simulink model "VehicleDynamicsModel"  (R2018a)
settings: Solver=ode15s  StartTime=0.0  StopTime=12  FixedStep=0.01  RelTol=1e-2  EnableMultiTasking=on
PreLoadFcn:
  | PowerTrain_14DOF_ini
StopFcn:
  | AfterSim
undefined symbols (not defined in the file): AccelCmd2TrqCmd, Chasis, GearRatio, Motor, Motor_J, Motor_RotorDamping, VEH, X, Y, Z
libraries: sm_lib x186, autolibutils x40, nesl_utility x23, vehdynlibtire x4, fuzblock x3, sharedtransform x2, autolibmappedmotorcommon x2, vehdynlibeom x1, vehdynlibsuspension x1, simulink x1, vehdynlibsteering x1
(part 7 of 11)

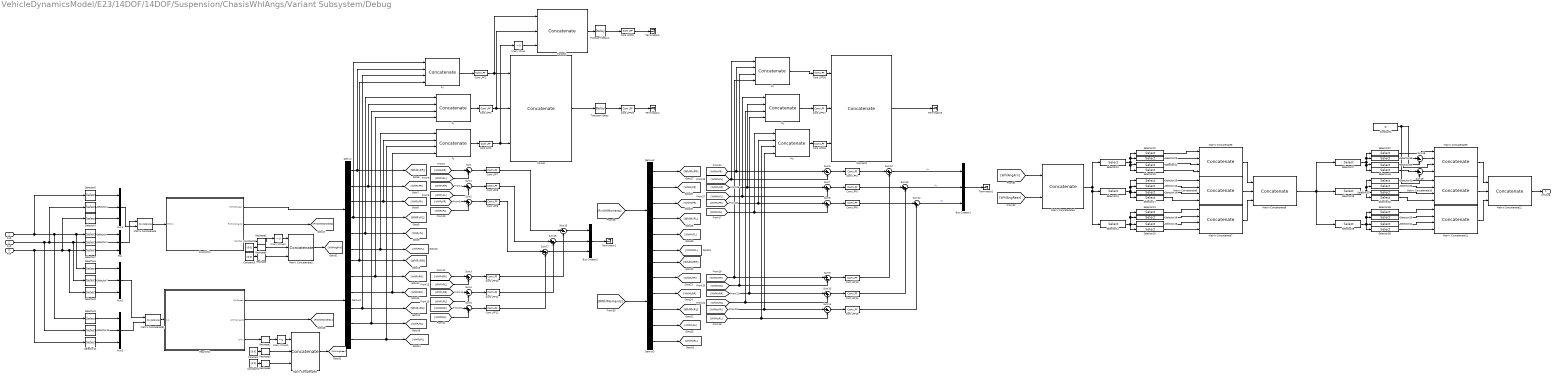
== system VehicleDynamicsModel/E23/14DOF/14DOF/Suspension/ChasisWhlAngs/Variant Subsystem/Debug ==
  FxR : Inport
  FyR : Inport  Port=2
  FzR : Inport  Port=3
  Bus Creator1 : BusCreator  Inputs=3
  Bus Creator2 : BusCreator  Inputs=3
  Constant{,1..3} (4 alike) : Constant  Value=[0 0]
  Constant4 : Constant  Value=pi
  Cont LPF{1..20} (20 alike) : autolibutils/Cont LPF  wc=2*pi  aMode=2
      settings: SourceProductName=Powertrain Blockset  SourceProductBaseCode=PW
  Demux{,1..3} (4 alike) : Demux  Outputs=6
  Forces : Concatenate  NumInputs=3  Mode=Multidimensional array
  Forces1 : Concatenate  NumInputs=3  Mode=Multidimensional array
  FrontWhls : Subsystem  TreatAsAtomicUnit=on
  Fx : Concatenate  NumInputs=4  Mode=Multidimensional array  ConcatenateDimension=2
  Fy : Concatenate  NumInputs=4  Mode=Multidimensional array  ConcatenateDimension=2
  Fz : Concatenate  NumInputs=4  Mode=Multidimensional array  ConcatenateDimension=2
  Matrix Concatenate : Concatenate  Mode=Multidimensional array  ConcatenateDimension=2
  Matrix Concatenate1 : Concatenate  Mode=Multidimensional array  ConcatenateDimension=2
  Matrix Concatenate{5..7,9..11} (6 alike) : Concatenate  NumInputs=4  Mode=Multidimensional array  ConcatenateDimension=2
  Matrix Concatenate{2..3,8,12} (4 alike) : Concatenate  NumInputs=3  Mode=Multidimensional array
  Matrix Concatenate4 : Concatenate  Mode=Multidimensional array  ConcatenateDimension=2
  Moments : Concatenate  NumInputs=3  Mode=Multidimensional array
  Mux{,1..3} (4 alike) : Mux  Inputs=3
  Mx : Concatenate  NumInputs=4  Mode=Multidimensional array  ConcatenateDimension=2
  My : Concatenate  NumInputs=4  Mode=Multidimensional array  ConcatenateDimension=2
  Mz : Concatenate  NumInputs=4  Mode=Multidimensional array  ConcatenateDimension=2
  RearWhls : Subsystem  TreatAsAtomicUnit=on
  Reshape{,1..5} (6 alike) : Reshape  OutputDimensionality=Row vector (2-D)
  Selector{,1..2,21..22,26,36..37,41} (9 alike) : Selector  InputPortWidth=4  IndexOptions=Index vector (dialog)  Indices=1  OutputSizes=1
  Selector{9..11,17,20,25,32,35,40} (9 alike) : Selector  InputPortWidth=4  IndexOptions=Index vector (dialog)  Indices=4  OutputSizes=1
  Selector12 : Selector  NumberOfDimensions=2  InputPortWidth=3  IndexOptions=Index vector (dialog),Select all  Indices=1,1  OutputSizes=1,1
  Selector13 : Selector  NumberOfDimensions=2  InputPortWidth=3  IndexOptions=Index vector (dialog),Select all  Indices=2,1  OutputSizes=1,1
  Selector14 : Selector  NumberOfDimensions=2  InputPortWidth=3  IndexOptions=Index vector (dialog),Select all  Indices=3,1  OutputSizes=1,1
  Selector{3..5,15,18,23,30,33,38} (9 alike) : Selector  InputPortWidth=4  IndexOptions=Index vector (dialog)  Indices=2  OutputSizes=1
  Selector{6..8,16,19,24,31,34,39} (9 alike) : Selector  InputPortWidth=4  IndexOptions=Index vector (dialog)  Indices=3  OutputSizes=1
  Selector27 : Selector  NumberOfDimensions=2  InputPortWidth=3  IndexOptions=Index vector (dialog),Select all  Indices=1,1  OutputSizes=1,1
  Selector28 : Selector  NumberOfDimensions=2  InputPortWidth=3  IndexOptions=Index vector (dialog),Select all  Indices=2,1  OutputSizes=1,1
  Selector29 : Selector  NumberOfDimensions=2  InputPortWidth=3  IndexOptions=Index vector (dialog),Select all  Indices=3,1  OutputSizes=1,1
  Sum{,2..3,5,7,10,12..14,16..17} (11 alike) : Sum  Inputs=|++
  Sum{1,4,6,8..9,11,15,18..19} (9 alike) : Sum  Inputs=|+-
  Terminator{1..5} (5 alike) : Terminator
  Transport Delay : TransportDelay  DelayTime=0
  Transport Delay1 : TransportDelay  DelayTime=0
  Unary Minus : UnaryMinus
  Unary Minus1 : UnaryMinus
  Unary Minus2 : UnaryMinus
  WhlAng : Outport
  wires:
  Matrix Concatenate7/1 -> Matrix Concatenate8/3
  Matrix Concatenate5/1 -> Matrix Concatenate8/1
  FyR/1 -> Selector10/1, Selector4/1, Selector7/1, Selector1/1
  FzR/1 -> Selector11/1, Selector3/1, Selector8/1, Selector2/1
  Selector17/1 -> Matrix Concatenate6/4
  Selector16/1 -> Matrix Concatenate6/3
  Matrix Concatenate4/1 -> Selector14/1, Selector13/1, Selector12/1
  Selector15/1 -> Matrix Concatenate6/2
  Selector21/1 -> Matrix Concatenate7/1
  Matrix Concatenate8/1 -> Selector29/1, Selector27/1, Selector28/1
  Selector40/1 -> Sum19/1
  Selector39/1 -> Matrix Concatenate9/3
  Sum19/1 -> Matrix Concatenate9/4
  Selector13/1 -> Selector15/1, Selector26/1, Selector17/1, Selector16/1
  Selector12/1 -> Selector25/1, Selector24/1, Selector23/1, Selector22/1
  Selector14/1 -> Selector20/1, Selector19/1, Selector18/1, Selector21/1
  Selector22/1 -> Matrix Concatenate5/1
  Selector37/1 -> Matrix Concatenate9/1
  Matrix Concatenate11/1 -> Matrix Concatenate12/3
  Selector36/1 -> Matrix Concatenate11/1
  Selector28/1 -> Selector30/1, Selector41/1, Selector32/1, Selector31/1
  Selector38/1 -> Sum18/1
  Selector27/1 -> Selector40/1, Selector39/1, Selector38/1, Selector37/1
  Matrix Concatenate10/1 -> Matrix Concatenate12/2
  Selector31/1 -> Matrix Concatenate10/3
  Selector32/1 -> Matrix Concatenate10/4
  Matrix Concatenate9/1 -> Matrix Concatenate12/1
  Constant4/1 -> Sum19/2, Sum18/2
  Selector34/1 -> Matrix Concatenate11/3
  Selector30/1 -> Matrix Concatenate10/2
  Sum18/1 -> Matrix Concatenate9/2
  Matrix Concatenate12/1 -> WhlAng/1
  [WhlMzRL] -> Mz/3, Sum11/2
  [WhlMxRL] -> Mx/3, Sum9/2
  [RWhlMoments] -> Demux3/1
  Demux1/2 -> Fy/4, [WhlFyRR]
  [WhlMyFL] -> My/1, Sum7/2
  Bus Creator2/1 -> Terminator1/1
  Mux2/1 -> Matrix Concatenate1/1
  Cont LPF6/1 -> Sum14/1
  Demux2/5 -> [WhlMyFL]
  [WhlMxFR] -> Mx/2, Sum6/1
  Selector33/1 -> Matrix Concatenate11/2
  My/1 -> Cont LPF17/1
  [WhlMyFR] -> My/2, Sum7/1
  Demux1/3 -> Fz/4, [WhlFzRR]
  Sum2/1 -> Cont LPF9/1
  Selector4/1 -> Mux1/2
  Demux/4 -> Fx/1, [WhlFxFL]
  Sum7/1 -> Cont LPF5/1
  Demux2/1 -> [WhlMxFR]
  RearWhls/1(WhlForces) -> Demux1/1
  Fy/1 -> Cont LPF1/1
  Matrix Concatenate1/1 -> RearWhls/1(In1)
  Demux3/2 -> [WhlMyRR]
  Moments/1 -> Terminator5/1
  Demux3/1 -> [WhlMxRR]
  [WhlFxRL] -> Sum3/2
  Reshape/1 -> Matrix Concatenate2/3
  Demux1/5 -> Fy/3, [WhlFyRL]
  FrontWhls/1(FWhlsForces) -> Demux/1
  [WhlFzFR] -> Sum2/1
  Demux2/6 -> [WhlMzFL]
  Cont LPF11/1 -> Sum16/2
  Sum1/1 -> Cont LPF8/1
  Cont LPF8/1 -> Sum16/1
  Demux1/1 -> Fx/4, [WhlFxRR]
  Sum17/1 -> Bus Creator2/3
  [WhlFyRL] -> Sum4/2
  [WhlMyRL] -> My/3, Sum10/2
  Selector24/1 -> Matrix Concatenate5/3
  Selector6/1 -> Mux2/1
  Cont LPF1/1 -> Forces1/2, Forces/2
  Cont LPF10/1 -> Sum15/2
  Demux3/4 -> [WhlMxRL]
  Cont LPF3/1 -> Unary Minus/1, Forces/3
  Cont LPF7/1 -> Sum15/1
  Cont LPF15/1 -> Sum14/2
  Sum4/1 -> Cont LPF11/1
  Mx/1 -> Cont LPF16/1
  [WhlFyFR] -> Sum1/1
  [WhlFzRR] -> Sum5/1
  Mux3/1 -> Matrix Concatenate1/2
  Cont LPF17/1 -> Moments/2
  Sum5/1 -> Cont LPF12/1
  Cont LPF2/1 -> Forces1/1, Forces/1
  [WhlFyRR] -> Sum4/1
  Selector26/1 -> Matrix Concatenate6/1
  Selector10/1 -> Mux3/2
  Unary Minus/1 -> Forces1/3
  [WhlFxRR] -> Sum3/1
  Forces/1 -> Transport Delay/1
  Transport Delay/1 -> Cont LPF19/1
  Selector8/1 -> Mux2/3
  Demux2/2 -> [WhlMyFR]
  Reshape4/1 -> Matrix Concatenate2/2
  Sum10/1 -> Cont LPF14/1
  Matrix Concatenate3/1 -> [WhlAngRear]
  Cont LPF9/1 -> Sum17/1
  [WhlAngFrn] -> Matrix Concatenate4/1
  Sum14/1 -> Bus Creator1/3  "Mz"
  Cont LPF19/1 -> Terminator4/1
  Cont LPF20/1 -> Terminator3/1
  Cont LPF16/1 -> Moments/1
  Demux/5 -> Fy/1, [WhlFyFL]
  Selector29/1 -> Selector35/1, Selector34/1, Selector33/1, Selector36/1
  RearWhls/2(WhlMoments) -> [RWhlMoments]
  Selector1/1 -> Mux/2
  Mux/1 -> Matrix Concatenate/1
  [WhlMxFL] -> Sum6/2, Mx/1
  [WhlFxFL] -> Sum/2
  Selector5/1 -> Mux1/1
  Constant/1 -> Reshape3/1
  Matrix Concatenate/1 -> FrontWhls/1(FWhls)
  Cont LPF5/1 -> Sum13/1
  Demux2/4 -> [WhlMxFL]
  Sum8/1 -> Cont LPF6/1
  Demux3/3 -> [WhlMzRR]
  Selector9/1 -> Mux3/1
  Selector11/1 -> Mux3/3
  Mux1/1 -> Matrix Concatenate/2
  Reshape2/1 -> Unary Minus1/1
  [WhlFzRL] -> Sum5/2
  Demux1/6 -> Fz/3, [WhlFzRL]
  Bus Creator1/1 -> Terminator2/1
  Selector23/1 -> Matrix Concatenate5/2
  Selector35/1 -> Matrix Concatenate11/4
  Constant3/1 -> Reshape/1
  RearWhls/3(Whl1) -> Reshape2/1
  Constant2/1 -> Reshape4/1
  Reshape5/1 -> Matrix Concatenate3/3
  Reshape3/1 -> Matrix Concatenate3/2
  Demux2/3 -> [WhlMzFR]
  Selector20/1 -> Matrix Concatenate7/4
  Selector18/1 -> Matrix Concatenate7/2
  Forces1/1 -> Transport Delay1/1
  Constant1/1 -> Reshape5/1
  FrontWhls/2(FWhlMoments) -> [FrnWhlMoments]
  Sum/1 -> Cont LPF7/1
  Demux3/6 -> [WhlMzRL]
  FrontWhls/3(Camber) -> Reshape1/1
  Reshape1/1 -> Unary Minus2/1
  Unary Minus1/1 -> Matrix Concatenate3/1
  Selector3/1 -> Mux1/3
  Demux3/5 -> [WhlMyRL]
  Selector41/1 -> Matrix Concatenate10/1
  Sum13/1 -> Bus Creator1/2  "My"
  Selector19/1 -> Matrix Concatenate7/3
  [WhlMzRR] -> Mz/4, Sum11/1
  Matrix Concatenate2/1 -> [WhlAngFrn]
  Cont LPF12/1 -> Sum17/2
  Cont LPF13/1 -> Sum12/2
  [WhlMzFR] -> Mz/2, Sum8/1
  Demux/3 -> Fz/2, [WhlFzFR]
  Demux/1 -> Fx/2, [WhlFxFR]
  [FrnWhlMoments] -> Demux2/1
  Demux/2 -> Fy/2, [WhlFyFR]
  Sum11/1 -> Cont LPF15/1
  Cont LPF18/1 -> Moments/3
  Sum12/1 -> Bus Creator1/1  "Mx"
  Sum15/1 -> Bus Creator2/1
  Cont LPF14/1 -> Sum13/2
  Fz/1 -> Cont LPF3/1
  Transport Delay1/1 -> Cont LPF20/1
  Sum9/1 -> Cont LPF13/1
  [WhlMxRR] -> Mx/4, Sum9/1
  Mz/1 -> Cont LPF18/1
  [WhlAngRear] -> Matrix Concatenate4/2
  [WhlMzFL] -> Mz/1, Sum8/2
  [WhlFzFL] -> Sum2/2
  [WhlFxFR] -> Sum/1
  Fx/1 -> Cont LPF2/1
  Selector/1 -> Mux/1
  Selector7/1 -> Mux2/2
  [WhlFyFL] -> Sum1/2
  Sum3/1 -> Cont LPF10/1
  Demux1/4 -> Fx/3, [WhlFxRL]
  Matrix Concatenate6/1 -> Matrix Concatenate8/2
  Selector2/1 -> Mux/3
  Sum16/1 -> Bus Creator2/2
  [WhlMyRR] -> My/4, Sum10/1
  Sum6/1 -> Cont LPF4/1
  Unary Minus2/1 -> Matrix Concatenate2/1
  Selector25/1 -> Matrix Concatenate5/4
  Demux/6 -> Fz/1, [WhlFzFL]
  Cont LPF4/1 -> Sum12/1
  FxR/1 -> Selector5/1, Selector9/1, Selector6/1, Selector/1

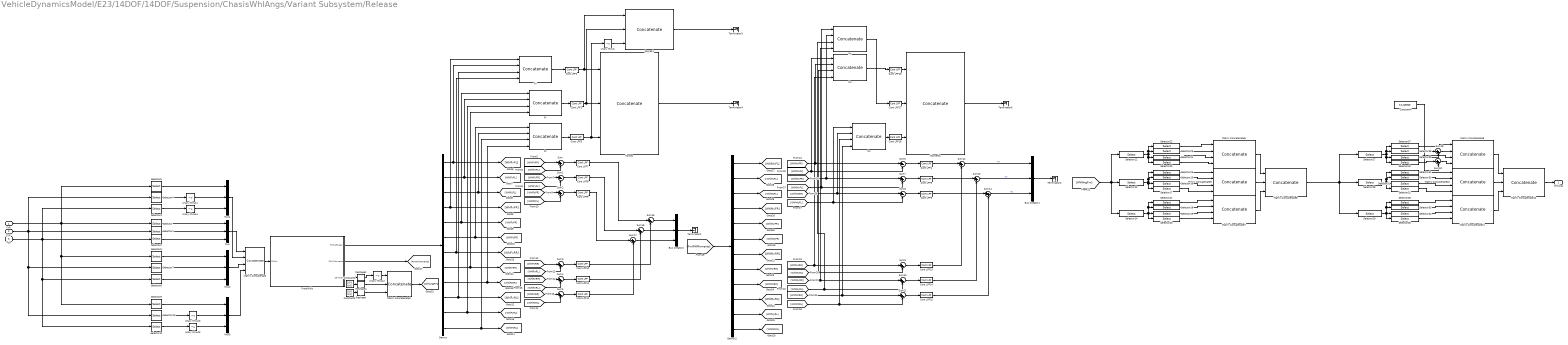
== system VehicleDynamicsModel/E23/14DOF/14DOF/Suspension/ChasisWhlAngs/Variant Subsystem/Release ==
  FxR : Inport
  FyR : Inport  Port=2
  FzR : Inport  Port=3
  Bus Creator1 : BusCreator  Inputs=3
  Bus Creator2 : BusCreator  Inputs=3
  Constant2 : Constant  Value=[0 0 0 0]
  Constant3 : Constant  Value=[0 0 0 0]
  Constant4 : Constant  Value=3.1415926
  Cont LPF{1..18} (18 alike) : autolibutils/Cont LPF  wc=2*pi  aMode=2
      settings: SourceProductName=Powertrain Blockset  SourceProductBaseCode=PW
  Demux : Demux  Outputs=12
  Demux2 : Demux  Outputs=12
  Forces : Concatenate  NumInputs=3  Mode=Multidimensional array
  Forces1 : Concatenate  NumInputs=3  Mode=Multidimensional array
  FrontWhls : Subsystem  TreatAsAtomicUnit=on
  Fx : Concatenate  NumInputs=4  Mode=Multidimensional array  ConcatenateDimension=2
  Fy : Concatenate  NumInputs=4  Mode=Multidimensional array  ConcatenateDimension=2
  Fz : Concatenate  NumInputs=4  Mode=Multidimensional array  ConcatenateDimension=2
  Matrix Concatenate{,5..7,9..11} (7 alike) : Concatenate  NumInputs=4  Mode=Multidimensional array  ConcatenateDimension=2
  Matrix Concatenate12 : Concatenate  NumInputs=3  Mode=Multidimensional array
  Matrix Concatenate2 : Concatenate  NumInputs=3  Mode=Multidimensional array
  Matrix Concatenate8 : Concatenate  NumInputs=3  Mode=Multidimensional array
  Moments : Concatenate  NumInputs=3  Mode=Multidimensional array
  Mux{,1..3} (4 alike) : Mux  Inputs=3
  Mx : Concatenate  NumInputs=4  Mode=Multidimensional array  ConcatenateDimension=2
  My : Concatenate  NumInputs=4  Mode=Multidimensional array  ConcatenateDimension=2
  Mz : Concatenate  NumInputs=4  Mode=Multidimensional array  ConcatenateDimension=2
  Reshape : Reshape  OutputDimensionality=Row vector (2-D)
  Reshape1 : Reshape  OutputDimensionality=Row vector (2-D)
  Reshape4 : Reshape  OutputDimensionality=Row vector (2-D)
  Selector{,1..2,21..22,26,36..37,41} (9 alike) : Selector  InputPortWidth=4  IndexOptions=Index vector (dialog)  Indices=1  OutputSizes=1
  Selector{9..11,17,20,25,32,35,40} (9 alike) : Selector  InputPortWidth=4  IndexOptions=Index vector (dialog)  Indices=4  OutputSizes=1
  Selector12 : Selector  NumberOfDimensions=2  InputPortWidth=3  IndexOptions=Index vector (dialog),Select all  Indices=1,1  OutputSizes=1,1
  Selector13 : Selector  NumberOfDimensions=2  InputPortWidth=3  IndexOptions=Index vector (dialog),Select all  Indices=2,1  OutputSizes=1,1
  Selector14 : Selector  NumberOfDimensions=2  InputPortWidth=3  IndexOptions=Index vector (dialog),Select all  Indices=3,1  OutputSizes=1,1
  Selector{3..5,15,18,23,30,33,38} (9 alike) : Selector  InputPortWidth=4  IndexOptions=Index vector (dialog)  Indices=2  OutputSizes=1
  Selector{6..8,16,19,24,31,34,39} (9 alike) : Selector  InputPortWidth=4  IndexOptions=Index vector (dialog)  Indices=3  OutputSizes=1
  Selector27 : Selector  NumberOfDimensions=2  InputPortWidth=3  IndexOptions=Index vector (dialog),Select all  Indices=1,1  OutputSizes=1,1
  Selector28 : Selector  NumberOfDimensions=2  InputPortWidth=3  IndexOptions=Index vector (dialog),Select all  Indices=2,1  OutputSizes=1,1
  Selector29 : Selector  NumberOfDimensions=2  InputPortWidth=3  IndexOptions=Index vector (dialog),Select all  Indices=3,1  OutputSizes=1,1
  Sum{,2..3,5,7,10,12..14,16..17} (11 alike) : Sum  Inputs=|++
  Sum{1,4,6,8..9,11,15,18..19} (9 alike) : Sum  Inputs=|+-
  Terminator{1..5} (5 alike) : Terminator
  Unary Minus{,1..5} (6 alike) : UnaryMinus
  WhlAng : Outport
  wires:
  Matrix Concatenate7/1 -> Matrix Concatenate8/3
  Matrix Concatenate5/1 -> Matrix Concatenate8/1
  FyR/1 -> Selector7/1, Selector10/1, Selector1/1, Selector4/1
  FzR/1 -> Selector3/1, Selector11/1, Selector8/1, Selector2/1
  Selector17/1 -> Matrix Concatenate6/4
  Selector16/1 -> Matrix Concatenate6/3
  [WhlAngFrn] -> Selector12/1, Selector14/1, Selector13/1
  Selector15/1 -> Matrix Concatenate6/2
  Selector21/1 -> Matrix Concatenate7/1
  Matrix Concatenate8/1 -> Selector29/1, Selector27/1, Selector28/1
  Selector13/1 -> Selector15/1, Selector26/1, Selector17/1, Selector16/1
  Selector12/1 -> Selector25/1, Selector24/1, Selector23/1, Selector22/1
  Selector14/1 -> Selector20/1, Selector19/1, Selector18/1, Selector21/1
  Selector22/1 -> Matrix Concatenate5/1
  Selector37/1 -> Matrix Concatenate9/1
  Matrix Concatenate11/1 -> Matrix Concatenate12/3
  Selector36/1 -> Matrix Concatenate11/1
  Selector28/1 -> Selector30/1, Selector41/1, Selector32/1, Selector31/1
  Selector38/1 -> Sum18/1
  Selector27/1 -> Selector40/1, Selector39/1, Selector38/1, Selector37/1
  Matrix Concatenate10/1 -> Matrix Concatenate12/2
  Selector31/1 -> Matrix Concatenate10/3
  Selector32/1 -> Matrix Concatenate10/4
  Matrix Concatenate9/1 -> Matrix Concatenate12/1
  Constant4/1 -> Sum18/2, Sum19/2
  Selector34/1 -> Matrix Concatenate11/3
  Selector30/1 -> Matrix Concatenate10/2
  Sum18/1 -> Matrix Concatenate9/2
  Matrix Concatenate12/1 -> WhlAng/1
  [WhlMzRL] -> Mz/3, Sum11/2
  [WhlMxRL] -> Mx/3, Sum9/2
  Demux/8 -> Fy/4, [WhlFyRR]
  [WhlMyFL] -> My/1, Sum7/2
  Bus Creator2/1 -> Terminator1/1
  Mux2/1 -> Matrix Concatenate/3
  Cont LPF6/1 -> Sum14/1
  Demux2/5 -> [WhlMyFR]
  [WhlMxFR] -> Mx/2, Sum6/1
  Selector33/1 -> Matrix Concatenate11/2
  My/1 -> Cont LPF17/1
  [WhlMyFR] -> My/2, Sum7/1
  Demux/9 -> Fz/4, [WhlFzRR]
  Sum2/1 -> Cont LPF9/1
  Selector4/1 -> Unary Minus1/1
  Demux/4 -> Fx/1, [WhlFxFR]
  Sum7/1 -> Cont LPF5/1
  Demux2/1 -> [WhlMxFL]
  Fy/1 -> Cont LPF1/1
  Demux2/8 -> [WhlMyRR]
  Moments/1 -> Terminator5/1
  Demux2/7 -> [WhlMxRR]
  [WhlFxRL] -> Sum3/2
  Reshape/1 -> Matrix Concatenate2/3
  Demux/11 -> Fy/3, [WhlFyRL]
  FrontWhls/1(FWhlsForces) -> Demux/1
  [WhlFzFR] -> Sum2/1
  Demux2/6 -> [WhlMzFR]
  Cont LPF11/1 -> Sum16/2
  Sum1/1 -> Cont LPF8/1
  Cont LPF8/1 -> Sum16/1
  Demux/7 -> Fx/4, [WhlFxRR]
  Sum17/1 -> Bus Creator2/3
  [WhlFyRL] -> Sum4/2
  [WhlMyRL] -> My/3, Sum10/2
  Selector24/1 -> Matrix Concatenate5/3
  Selector6/1 -> Mux2/1
  Cont LPF1/1 -> Forces1/2, Forces/2
  Cont LPF10/1 -> Sum15/2
  Demux2/10 -> [WhlMxRL]
  Cont LPF3/1 -> Unary Minus/1, Forces/3
  Cont LPF7/1 -> Sum15/1
  Cont LPF15/1 -> Sum14/2
  Sum4/1 -> Cont LPF11/1
  Mx/1 -> Cont LPF16/1
  [WhlFyFR] -> Sum1/1
  [WhlFzRR] -> Sum5/1
  Mux3/1 -> Matrix Concatenate/4
  Cont LPF17/1 -> Moments/2
  Sum5/1 -> Cont LPF12/1
  Cont LPF2/1 -> Forces1/1, Forces/1
  [WhlFyRR] -> Sum4/1
  Selector26/1 -> Matrix Concatenate6/1
  Unary Minus/1 -> Forces1/3
  [WhlFxRR] -> Sum3/1
  Demux2/2 -> [WhlMyFL]
  Reshape4/1 -> Matrix Concatenate2/2
  Sum10/1 -> Cont LPF14/1
  Cont LPF9/1 -> Sum17/1
  Sum14/1 -> Bus Creator1/3  "Mz"
  Forces/1 -> Terminator4/1
  Forces1/1 -> Terminator3/1
  Cont LPF16/1 -> Moments/1
  Demux/5 -> Fy/1, [WhlFyFR]
  Selector29/1 -> Selector35/1, Selector34/1, Selector33/1, Selector36/1
  [WhlMxFL] -> Sum6/2, Mx/1
  [WhlFxFL] -> Sum/2
  Matrix Concatenate/1 -> FrontWhls/1(FWhls)
  Cont LPF5/1 -> Sum13/1
  Demux2/4 -> [WhlMxFR]
  Sum8/1 -> Cont LPF6/1
  Demux2/9 -> [WhlMzRR]
  Selector9/1 -> Mux3/1
  [WhlFzRL] -> Sum5/2
  Demux/12 -> Fz/3, [WhlFzRL]
  Bus Creator1/1 -> Terminator2/1
  Selector23/1 -> Matrix Concatenate5/2
  Selector35/1 -> Matrix Concatenate11/4
  Constant3/1 -> Reshape/1
  Constant2/1 -> Reshape4/1
  Demux2/3 -> [WhlMzFL]
  Selector20/1 -> Matrix Concatenate7/4
  Selector18/1 -> Matrix Concatenate7/2
  FrontWhls/2(FWhlMoments) -> [FrnWhlMoments]
  Sum/1 -> Cont LPF7/1
  Demux2/12 -> [WhlMzRL]
  Reshape1/1 -> Unary Minus2/1
  Demux2/11 -> [WhlMyRL]
  Selector41/1 -> Matrix Concatenate10/1
  Sum13/1 -> Bus Creator1/2  "My"
  Selector19/1 -> Matrix Concatenate7/3
  [WhlMzRR] -> Mz/4, Sum11/1
  Matrix Concatenate2/1 -> [WhlAngFrn]
  Cont LPF12/1 -> Sum17/2
  Cont LPF13/1 -> Sum12/2
  [WhlMzFR] -> Mz/2, Sum8/1
  Demux/3 -> Fz/2, [WhlFzFL]
  Demux/1 -> Fx/2, [WhlFxFL]
  [FrnWhlMoments] -> Demux2/1
  Demux/2 -> Fy/2, [WhlFyFL]
  Sum11/1 -> Cont LPF15/1
  Cont LPF18/1 -> Moments/3
  Sum12/1 -> Bus Creator1/1  "Mx"
  Sum15/1 -> Bus Creator2/1
  Cont LPF14/1 -> Sum13/2
  Fz/1 -> Cont LPF3/1
  Sum9/1 -> Cont LPF13/1
  [WhlMxRR] -> Mx/4, Sum9/1
  Mz/1 -> Cont LPF18/1
  [WhlMzFL] -> Mz/1, Sum8/2
  [WhlFzFL] -> Sum2/2
  [WhlFxFR] -> Sum/1
  Fx/1 -> Cont LPF2/1
  Selector/1 -> Mux/1
  Selector7/1 -> Mux2/2
  [WhlFyFL] -> Sum1/2
  Sum3/1 -> Cont LPF10/1
  Demux/10 -> Fx/3, [WhlFxRL]
  Matrix Concatenate6/1 -> Matrix Concatenate8/2
  Sum16/1 -> Bus Creator2/2
  [WhlMyRR] -> Sum10/1, My/4
  Sum6/1 -> Cont LPF4/1
  Unary Minus2/1 -> Matrix Concatenate2/1
  Selector25/1 -> Matrix Concatenate5/4
  Demux/6 -> Fz/1, [WhlFzFR]
  Cont LPF4/1 -> Sum12/1
  FxR/1 -> Selector6/1, Selector9/1, Selector/1, Selector5/1
  Selector39/1 -> Matrix Concatenate9/3
  Selector40/1 -> Sum19/1
  Sum19/1 -> Matrix Concatenate9/4
  Mux/1 -> Matrix Concatenate/1
  Mux1/1 -> Matrix Concatenate/2
  Selector5/1 -> Mux1/1
  Selector3/1 -> Unary Minus4/1
  Selector8/1 -> Mux2/3
  Selector11/1 -> Unary Minus5/1
  Selector2/1 -> Mux/3
  FrontWhls/3(Camber) -> Reshape1/1
  Selector10/1 -> Unary Minus3/1
  Selector1/1 -> Mux/2
  Unary Minus3/1 -> Mux3/2
  Unary Minus1/1 -> Mux1/2
  Unary Minus4/1 -> Mux1/3
  Unary Minus5/1 -> Mux3/3

== system VehicleDynamicsModel/E23/14DOF/14DOF/Tires&Wheels/VDBS/4Wheels/Fx ==
  In1 : Inport
  In2 : Inport  Port=2
  In3 : Inport  Port=3
  In4 : Inport  Port=4
  Bus Selector{,1..3} (4 alike) : BusSelector  OutputSignals=Fx
  Vector Concatenate : Concatenate  NumInputs=4
  Fx : Outport
  wires:
  Bus Selector/1 -> Vector Concatenate/1  "<Fx>"
  Bus Selector1/1 -> Vector Concatenate/2  "<Fx>"
  In2/1 -> Bus Selector1/1
  Vector Concatenate/1 -> Fx/1
  Bus Selector3/1 -> Vector Concatenate/4  "<Fx>"
  In3/1 -> Bus Selector2/1
  In4/1 -> Bus Selector3/1
  Bus Selector2/1 -> Vector Concatenate/3  "<Fx>"
  In1/1 -> Bus Selector/1

== system VehicleDynamicsModel/E23/14DOF/14DOF/Tires&Wheels/VDBS/4Wheels/Fy ==
  In1 : Inport
  In2 : Inport  Port=2
  In3 : Inport  Port=3
  In4 : Inport  Port=4
  Bus Selector{,1..3} (4 alike) : BusSelector  OutputSignals=Fy
  Vector Concatenate : Concatenate  NumInputs=4
  Fy : Outport
  wires:
  Bus Selector/1 -> Vector Concatenate/1  "<Fy>"
  Bus Selector1/1 -> Vector Concatenate/2  "<Fy>"
  In2/1 -> Bus Selector1/1
  Vector Concatenate/1 -> Fy/1
  Bus Selector3/1 -> Vector Concatenate/4  "<Fy>"
  In3/1 -> Bus Selector2/1
  In4/1 -> Bus Selector3/1
  Bus Selector2/1 -> Vector Concatenate/3  "<Fy>"
  In1/1 -> Bus Selector/1

== system VehicleDynamicsModel/E23/14DOF/14DOF/Tires&Wheels/VDBS/4Wheels/Fz ==
  In1 : Inport
  In2 : Inport  Port=2
  In3 : Inport  Port=3
  In4 : Inport  Port=4
  Bus Selector{,1..3} (4 alike) : BusSelector  OutputSignals=Fz
  Vector Concatenate : Concatenate  NumInputs=4
  Fz : Outport
  wires:
  Bus Selector/1 -> Vector Concatenate/1  "<Fz>"
  Bus Selector1/1 -> Vector Concatenate/2  "<Fz>"
  In2/1 -> Bus Selector1/1
  Vector Concatenate/1 -> Fz/1
  Bus Selector3/1 -> Vector Concatenate/4  "<Fz>"
  In3/1 -> Bus Selector2/1
  In4/1 -> Bus Selector3/1
  Bus Selector2/1 -> Vector Concatenate/3  "<Fz>"
  In1/1 -> Bus Selector/1

== system VehicleDynamicsModel/E23/14DOF/14DOF/Tires&Wheels/VDBS/4Wheels/Kappa ==
  In1 : Inport
  In2 : Inport  Port=2
  In3 : Inport  Port=3
  In4 : Inport  Port=4
  Bus Selector{,1..3} (4 alike) : BusSelector  OutputSignals=Kappa
  Vector Concatenate : Concatenate  NumInputs=4
  Kappa : Outport
  wires:
  Bus Selector/1 -> Vector Concatenate/1  "<Kappa>"
  Bus Selector1/1 -> Vector Concatenate/2  "<Kappa>"
  In2/1 -> Bus Selector1/1
  Vector Concatenate/1 -> Kappa/1
  Bus Selector3/1 -> Vector Concatenate/4  "<Kappa>"
  In3/1 -> Bus Selector2/1
  In4/1 -> Bus Selector3/1
  Bus Selector2/1 -> Vector Concatenate/3  "<Kappa>"
  In1/1 -> Bus Selector/1

== system VehicleDynamicsModel/E23/14DOF/14DOF/Tires&Wheels/VDBS/4Wheels/Mx ==
  In1 : Inport
  In2 : Inport  Port=2
  In3 : Inport  Port=3
  In4 : Inport  Port=4
  Bus Selector{,1..3} (4 alike) : BusSelector  OutputSignals=Mx
  Vector Concatenate : Concatenate  NumInputs=4
  Mx : Outport
  wires:
  Bus Selector/1 -> Vector Concatenate/1  "<Mx>"
  Bus Selector1/1 -> Vector Concatenate/2  "<Mx>"
  In2/1 -> Bus Selector1/1
  Vector Concatenate/1 -> Mx/1
  Bus Selector3/1 -> Vector Concatenate/4  "<Mx>"
  In3/1 -> Bus Selector2/1
  In4/1 -> Bus Selector3/1
  Bus Selector2/1 -> Vector Concatenate/3  "<Mx>"
  In1/1 -> Bus Selector/1

== system VehicleDynamicsModel/E23/14DOF/14DOF/Tires&Wheels/VDBS/4Wheels/My ==
  In1 : Inport
  In2 : Inport  Port=2
  In3 : Inport  Port=3
  In4 : Inport  Port=4
  Bus Selector{,1..3} (4 alike) : BusSelector  OutputSignals=My
  Vector Concatenate : Concatenate  NumInputs=4
  My : Outport
  wires:
  Bus Selector/1 -> Vector Concatenate/1  "<My>"
  Bus Selector1/1 -> Vector Concatenate/2  "<My>"
  In2/1 -> Bus Selector1/1
  Vector Concatenate/1 -> My/1
  Bus Selector3/1 -> Vector Concatenate/4  "<My>"
  In3/1 -> Bus Selector2/1
  In4/1 -> Bus Selector3/1
  Bus Selector2/1 -> Vector Concatenate/3  "<My>"
  In1/1 -> Bus Selector/1

== system VehicleDynamicsModel/E23/14DOF/14DOF/Tires&Wheels/VDBS/4Wheels/Mz ==
  In1 : Inport
  In2 : Inport  Port=2
  In3 : Inport  Port=3
  In4 : Inport  Port=4
  Bus Selector{,1..3} (4 alike) : BusSelector  OutputSignals=Mz
  Vector Concatenate : Concatenate  NumInputs=4
  Mz : Outport
  wires:
  Bus Selector/1 -> Vector Concatenate/1  "<Mz>"
  Bus Selector1/1 -> Vector Concatenate/2  "<Mz>"
  In2/1 -> Bus Selector1/1
  Vector Concatenate/1 -> Mz/1
  Bus Selector3/1 -> Vector Concatenate/4  "<Mz>"
  In3/1 -> Bus Selector2/1
  In4/1 -> Bus Selector3/1
  Bus Selector2/1 -> Vector Concatenate/3  "<Mz>"
  In1/1 -> Bus Selector/1

== system VehicleDynamicsModel/E23/14DOF/14DOF/Tires&Wheels/VDBS/4Wheels/Re ==
  In1 : Inport
  In2 : Inport  Port=2
  In3 : Inport  Port=3
  In4 : Inport  Port=4
  Bus Selector{,1..3} (4 alike) : BusSelector  OutputSignals=Re
  Vector Concatenate : Concatenate  NumInputs=4
  Re : Outport
  wires:
  Bus Selector/1 -> Vector Concatenate/1  "<Re>"
  Bus Selector1/1 -> Vector Concatenate/2  "<Re>"
  In2/1 -> Bus Selector1/1
  Vector Concatenate/1 -> Re/1
  Bus Selector3/1 -> Vector Concatenate/4  "<Re>"
  In3/1 -> Bus Selector2/1
  In4/1 -> Bus Selector3/1
  Bus Selector2/1 -> Vector Concatenate/3  "<Re>"
  In1/1 -> Bus Selector/1

== system VehicleDynamicsModel/E23/14DOF/14DOF/Tires&Wheels/VDBS/4Wheels/omega ==
  In1 : Inport
  In2 : Inport  Port=2
  In3 : Inport  Port=3
  In4 : Inport  Port=4
  Bus Selector{,1..3} (4 alike) : BusSelector  OutputSignals=Omega
  Vector Concatenate : Concatenate  NumInputs=4
  omege : Outport
  wires:
  Bus Selector/1 -> Vector Concatenate/1  "<Omega>"
  Bus Selector1/1 -> Vector Concatenate/2  "<Omega>"
  In2/1 -> Bus Selector1/1
  Vector Concatenate/1 -> omege/1
  Bus Selector3/1 -> Vector Concatenate/4  "<Omega>"
  In3/1 -> Bus Selector2/1
  In4/1 -> Bus Selector3/1
  Bus Selector2/1 -> Vector Concatenate/3  "<Omega>"
  In1/1 -> Bus Selector/1

== system VehicleDynamicsModel/E23/14DOF/14DOF/Tires&Wheels/VDBS/4Wheels/z ==
  In1 : Inport
  In2 : Inport  Port=2
  In3 : Inport  Port=3
  In4 : Inport  Port=4
  Bus Selector{,1..3} (4 alike) : BusSelector  OutputSignals=z
  Vector Concatenate : Concatenate  NumInputs=4
  Z : Outport
  wires:
  Bus Selector/1 -> Vector Concatenate/1  "<z>"
  Bus Selector1/1 -> Vector Concatenate/2  "<z>"
  In2/1 -> Bus Selector1/1
  Vector Concatenate/1 -> Z/1
  Bus Selector3/1 -> Vector Concatenate/4  "<z>"
  In3/1 -> Bus Selector2/1
  In4/1 -> Bus Selector3/1
  Bus Selector2/1 -> Vector Concatenate/3  "<z>"
  In1/1 -> Bus Selector/1

== system VehicleDynamicsModel/E23/14DOF/14DOF/Tires&Wheels/VDBS/4Wheels/zdot ==
  In1 : Inport
  In2 : Inport  Port=2
  In3 : Inport  Port=3
  In4 : Inport  Port=4
  Bus Selector{,1..3} (4 alike) : BusSelector  OutputSignals=zdot
  Vector Concatenate : Concatenate  NumInputs=4
  zdot : Outport
  wires:
  Bus Selector/1 -> Vector Concatenate/1  "<zdot>"
  Bus Selector1/1 -> Vector Concatenate/2  "<zdot>"
  In2/1 -> Bus Selector1/1
  Vector Concatenate/1 -> zdot/1
  Bus Selector3/1 -> Vector Concatenate/4  "<zdot>"
  In3/1 -> Bus Selector2/1
  In4/1 -> Bus Selector3/1
  Bus Selector2/1 -> Vector Concatenate/3  "<zdot>"
  In1/1 -> Bus Selector/1

== system VehicleDynamicsModel/E23/14DOF/14DOF/Tires&Wheels/VDBS/Tires2Veh/Subsystem ==
  note: 按行放置，即X ; Y ; Z
  note: 车轮坐标系
  note: 转向角（绕Z轴）
  note: 轮胎与车轮
      | 坐标系绕y轴
      | 角度为0
  note: 内倾角（绕X轴）
  Front : Inport
  Camber : Inport  Port=2
  Add : Sum
  Add1 : Sum
  Constant : Constant  Value=pi
  Constant1 : Constant  Value=[pi;0;pi;0].*0+[0;pi;0;pi].*.0
  Constant2 : Constant  Value=ones(1,4).*0
  Reshape : Reshape  OutputDimensionality=Row vector (2-D)
  Reshape1 : Reshape  OutputDimensionality=Row vector (2-D)
  Reshape2 : Reshape  OutputDimensionality=Row vector (2-D)
  Vector Concatenate1 : Concatenate  NumInputs=3  Mode=Multidimensional array
  Vehicle : Outport
  wires:
  Reshape/1 -> Vector Concatenate1/1
  Vector Concatenate1/1 -> Vehicle/1
  Add1/1 -> Reshape2/1
  Front/1 -> Add1/1
  Reshape1/1 -> Vector Concatenate1/2
  Constant1/1 -> Add1/2
  Reshape2/1 -> Vector Concatenate1/3
  Camber/1 -> Add/1
  Constant/1 -> Add/2
  Constant2/1 -> Reshape1/1
  Add/1 -> Reshape/1

== system VehicleDynamicsModel/E23/14DOF/14DOF/Tires&Wheels/VDBS/Tires2Veh/Subsystem1 ==
  Mx : Inport
  My : Inport  Port=2
  Mz : Inport  Port=3
  Re : Inport  Port=4
  z : Inport  Port=5
  zdot : Inport  Port=6
  Kappa : Inport  Port=7
  Fx : Inport  Port=8
  omega : Inport  Port=9
  Fy : Inport  Port=10
  Fz : Inport  Port=11
  Bus Creator : BusCreator  Inputs=11
  Reshape : Reshape  OutputDimensionality=Row vector (2-D)
  Reshape1 : Reshape  OutputDimensionality=Row vector (2-D)
  Unary Minus : UnaryMinus
  Unary Minus2 : UnaryMinus
  Whl : Outport
  zout : Outport  Port=2
  zdotout : Outport  Port=3
  wires:
  Mz/1 -> Bus Creator/7
  Fz/1 -> Bus Creator/4
  Fx/1 -> Bus Creator/2
  My/1 -> Bus Creator/6
  Fy/1 -> Bus Creator/3
  Re/1 -> Bus Creator/8
  omega/1 -> Bus Creator/1
  Mx/1 -> Bus Creator/5
  Unary Minus/1 -> Reshape1/1, Bus Creator/10  "zdot"
  Reshape1/1 -> zdotout/1
  Kappa/1 -> Bus Creator/11
  Bus Creator/1 -> Whl/1
  Reshape/1 -> zout/1
  Unary Minus2/1 -> Bus Creator/9, Reshape/1  "z"
  z/1 -> Unary Minus2/1  "z"
  zdot/1 -> Unary Minus/1

== system VehicleDynamicsModel/E23/14DOF/14DOF/Tires&Wheels/VDBS/Tires2Veh/WheeltoBodyTransform ==
  note: 矩阵相乘，把车轮坐标系下的力变换为车身坐标系下的力
  Forces : Inport  Partition=on  PartitionDimension=2  PartitionWidth=1  PartitionOffset=0
  WheelAngles : Inport  Port=2  Partition=on  PartitionDimension=2  PartitionWidth=1  PartitionOffset=0
  Demux : Demux  Outputs=3
  For Each : ForEach  DisableCoverage=on  IndexMode=One-based
  Matrix Multiply : Product  Multiplication=Matrix(*)
  Rotation Angles to Direction Cosine Matrix : sharedtransform/Rotation Angles to Direction Cosine Matrix  rotationOrder=ZYX  aMode=aMode
      settings: SourceProductBaseCode=AE
  Selector : Selector  InputPortWidth=3  IndexOptions=Index vector (dialog)  Indices=[3 2 1]  OutputSizes=1
  Fx : Outport  ConcatenationDimension=1
  Fy : Outport  Port=2  ConcatenationDimension=1
  Fz : Outport  Port=3  ConcatenationDimension=1
  wires:
  WheelAngles/1 -> Selector/1
  Selector/1 -> Rotation Angles to Direction Cosine Matrix/1
  Rotation Angles to Direction Cosine Matrix/1 -> Matrix Multiply/1
  Forces/1 -> Matrix Multiply/2
  Demux/1 -> Fx/1
  Matrix Multiply/1 -> Demux/1
  Demux/2 -> Fy/1
  Demux/3 -> Fz/1

== system VehicleDynamicsModel/E23/14DOF/14DOF/Tires&Wheels/VDBS/Veh2Tire/WheelAngles ==
  Camber : Inport
  Steer : Inport  Port=2
  Constant : Constant  Value=pi
  Constant2 : Constant  Value=[pi;0;pi;0].*0+[0;pi;0;pi].*0
  Reshape : Reshape  OutputDimensionality=Row vector (2-D)
  Reshape1 : Reshape  OutputDimensionality=Row vector (2-D)
  Reshape2 : Reshape  OutputDimensionality=Row vector (2-D)
  Vector Concatenate : Concatenate  NumInputs=3  Mode=Multidimensional array
  X : Sum
  Y : Constant  Value=ones(1,4).*0
  Z : Sum
  Vehicle : Outport
  wires:
  Y/1 -> Reshape1/1
  Reshape2/1 -> Vector Concatenate/3
  Constant/1 -> X/2
  Reshape1/1 -> Vector Concatenate/2
  Steer/1 -> Z/1
  Reshape/1 -> Vector Concatenate/1
  Vector Concatenate/1 -> Vehicle/1
  Camber/1 -> X/1
  Constant2/1 -> Z/2
  X/1 -> Reshape/1
  Z/1 -> Reshape2/1

== system VehicleDynamicsModel/E23/14DOF/14DOF/Tires&Wheels/VDBS/Veh2Tire/WheeltoBodyTransform ==
  note: 把车辆质心在车身坐标系下的速度转化为在车轮坐标系下的速度
  WheelAngles : Inport  Partition=on  PartitionDimension=2  PartitionWidth=1  PartitionOffset=0
  VelVeh : Inport  Port=2  Partition=on  PartitionDimension=2  PartitionWidth=1  PartitionOffset=0
  Demux : Demux  Outputs=3
  For Each : ForEach  DisableCoverage=on  IndexMode=One-based
  Matrix Multiply : Product  Multiplication=Matrix(*)
  Rotation Angles to Direction Cosine Matrix : sharedtransform/Rotation Angles to Direction Cosine Matrix  rotationOrder=ZYX  aMode=aMode
      settings: SourceProductBaseCode=AE
  Selector : Selector  InputPortWidth=3  IndexOptions=Index vector (dialog)  Indices=[3 2 1]  OutputSizes=1
  xdotWheel : Outport  ConcatenationDimension=1
  ydotWheel : Outport  Port=2  ConcatenationDimension=1
  zdotWheel : Outport  Port=3  ConcatenationDimension=1
  wires:
  WheelAngles/1 -> Selector/1
  Selector/1 -> Rotation Angles to Direction Cosine Matrix/1
  Rotation Angles to Direction Cosine Matrix/1 -> Matrix Multiply/1
  VelVeh/1 -> Matrix Multiply/2
  Matrix Multiply/1 -> Demux/1
  Demux/1 -> xdotWheel/1
  Demux/2 -> ydotWheel/1
  Demux/3 -> zdotWheel/1

== system VehicleDynamicsModel/E23/PowerTrain/PowerTrain/MotorRL/Motor/Motor/Mapped Motor ==
  BattVolt : Inport
  MtrSpd : Inport  Port=2
  TrqCmd : Inport  Port=3
  Mapped Motor Core Speed 4 : autolibmappedmotorcommon/Mapped Motor Core Speed 4
      settings: SourceProductName=Powertrain Blockset  SourceProductBaseCode=PW
  Info : Outport
  BattCurr : Outport  Port=2
  MtrTrq : Outport  Port=3
  wires:
  BattVolt/1 -> Mapped Motor Core Speed 4/1
  TrqCmd/1 -> Mapped Motor Core Speed 4/3
  MtrSpd/1 -> Mapped Motor Core Speed 4/2
  Mapped Motor Core Speed 4/2 -> BattCurr/1
  Mapped Motor Core Speed 4/1 -> Info/1
  Mapped Motor Core Speed 4/3 -> MtrTrq/1

== system VehicleDynamicsModel/E23/PowerTrain/PowerTrain/MotorRR/Motor/Motor/Mapped Motor ==
  BattVolt : Inport
  MtrSpd : Inport  Port=2
  TrqCmd : Inport  Port=3
  Mapped Motor Core Speed 4 : autolibmappedmotorcommon/Mapped Motor Core Speed 4
      settings: SourceProductName=Powertrain Blockset  SourceProductBaseCode=PW
  Info : Outport
  BattCurr : Outport  Port=2
  MtrTrq : Outport  Port=3
  wires:
  BattVolt/1 -> Mapped Motor Core Speed 4/1
  TrqCmd/1 -> Mapped Motor Core Speed 4/3
  MtrSpd/1 -> Mapped Motor Core Speed 4/2
  Mapped Motor Core Speed 4/2 -> BattCurr/1
  Mapped Motor Core Speed 4/1 -> Info/1
  Mapped Motor Core Speed 4/3 -> MtrTrq/1

== system VehicleDynamicsModel/E23/14DOF/14DOF/Suspension/ChasisWhlAngs/Variant Subsystem/Debug/FrontWhls ==
  FWhls : Inport  Partition=on  PartitionDimension=2  PartitionWidth=1  PartitionOffset=0
  Demux : Demux  Outputs=3
  External Force and Torque : sm_lib/Forces and Torques/External Force and Torque  ForceResolutionFrame=AttachedFrame  EnableForceX=on  EnableForceY=on  EnableForceZ=on  EnableForce=off  TorqueResolutionFrame=AttachedFrame  EnableTorqueX=off  EnableTorqueY=off  EnableTorqueZ=off  EnableTorque=off
  FR : Subsystem
  For Each : ForEach  DisableCoverage=on  IndexMode=One-based
  Frame : sm_lib/Body Elements/Solid  InertiaType=CalculateFromGeometry  Mass=1  MassUnits=kg  CenterOfMass=[0 0 0]  CenterOfMassUnits=m  MomentsOfInertia=[1 1 1]  MomentsOfInertiaUnits=kg*m^2  ProductsOfInertia=[0 0 0]  ProductsOfInertiaUnits=kg*m^2  DensityBased=off  Density=1000  DensityUnits=kg/m^3  DoExposeReferenceFrame=on  SerializedFrames=<Frames><Frame><Id>Frame1</Id><Value><Name>FR1</Name><Origin><Source>GeometricFeature</Source><FeatureName>planar surface 126</FeatureName></Origin><PrimaryAxis><DefinedDirection>+Z</DefinedDirection><Source>GeometricFeature</Source><SourceDirection>+Z</SourceDirection><FeatureName>segment 749</FeatureName></PrimaryAxis><SecondaryAxis><DefinedDirection>+X</DefinedDirection><Source>CenterOfMassFrame</Source><SourceDirection>+X</SourceDirection><FeatureName></FeatureName></SecondaryAxis></Value></Frame><Frame><Id>Frame2</Id><Value><Name>FR2</Name><Origin><Source>GeometricFeature</Source><FeatureName>planar surface 142</FeatureName></Origin><PrimaryAxis><DefinedDirection>+Y</DefinedDirection><Source>GeometricFeature</Source><SourceDirection>+Z</SourceDirection><FeatureName>planar surface 142</FeatureName></PrimaryAxis><SecondaryAxis><DefinedDirection>+Z</DefinedDirection><Source>CenterOfMassFrame</Source><SourceDirection>+X</SourceDirection><FeatureName></FeatureName></SecondaryAxis></Value></Frame><Frame><Id>Frame3</Id><Value><Name>FR3</Name><Origin><Source>GeometricFeature</Source><FeatureName>planar surface 180</FeatureName></Origin><PrimaryAxis><DefinedDirection>+X</DefinedDirection><Source>GeometricFeature</Source><SourceDirection>+Z</SourceDirection><FeatureName>planar surface 180</FeatureName></PrimaryAxis><SecondaryAxis><DefinedDirection>+Z</DefinedDirection><Source>ReferenceFrame</Source><SourceDirection>+X</SourceDirection><FeatureName></FeatureName></SecondaryAxis></Value></Frame><Frame><Id>Frame4</Id><Value><Name>FR4</Name><Origin><Source>GeometricFeature</Source><FeatureName>planar surface 188</FeatureName></Origin><PrimaryAxis><DefinedDirection>+Z</DefinedDirection><Source>GeometricFeature</Source><SourceDirection>+Z</SourceDirection><FeatureName>planar surface 188</FeatureName></PrimaryAxis><SecondaryAxis><DefinedDirection>+Y</DefinedDirection><Source>ReferenceFrame</Source><SourceDirection>+X</SourceDirection><FeatureName></FeatureName></SecondaryAxis></Value></Frame><Frame><Id>Frame5</Id><Value><Name>CoM</Name><Origin><Source>CenterOfMassFrame</Source><FeatureName></FeatureName></Origin><PrimaryAxis><DefinedDirection>+Z</DefinedDirection><Source>ReferenceFrame</Source><SourceDirection>+Z</SourceDirection><FeatureName></FeatureName></PrimaryAxis><SecondaryAxis><DefinedDirection>+X</DefinedDirection><Source>ReferenceFrame</Source><SourceDirection>+X</SourceDirection><FeatureName></FeatureName></SecondaryAxis></Value></Frame><Frame><Id>Frame6</Id><Value><Name>Frame_SwimArmFR</Name><Origin><Source>GeometricFeature</Source><FeatureName>circular curve 6</FeatureName></Origin><PrimaryAxis><DefinedDirection>+Z</DefinedDirection><Source>CenterOfMassFrame</Source><SourceDirection>+X</SourceDirection><FeatureName></FeatureName></PrimaryAxis><SecondaryAxis><DefinedDirection>+X</DefinedDirection><Source>CenterOfMassFrame</Source><SourceDirection>+Y</SourceDirection><FeatureName></FeatureName></SecondaryAxis></Value></Frame><Frame><Id>Frame7</Id><Value><Name>FL1</Name><Origin><Source>GeometricFeature</Source><FeatureName>planar surface 1</FeatureName></Origin><PrimaryAxis><DefinedDirection>-Z</DefinedDirection><Source>GeometricFeature</Source><SourceDirection>+Z</SourceDirection><FeatureName>segment 173</FeatureName></PrimaryAxis><SecondaryAxis><DefinedDirection>+X</DefinedDirection><Source>ReferenceFrame</Source><SourceDirection>+X</SourceDirection><FeatureName></FeatureName></SecondaryAxis></Value></Frame><Frame><Id>Frame8</Id><Value><Name>FL2</Name><Origin><Source>GeometricFeature</Source><FeatureName>planar surface 17</FeatureName></Origin><PrimaryAxis><DefinedDirection>-Y</DefinedDirection><Source>GeometricFeature</Source><SourceDirection>+Z</SourceDirection><FeatureName>planar surface 17</FeatureName></PrimaryAxis><SecondaryAxis><DefinedDirection>+Z</DefinedDirection><Source>CenterOfMassFrame</Source><SourceDirection>+X</SourceDirection><FeatureName></FeatureName></SecondaryAxis></Value></Frame><Frame><Id>Frame9</Id><Value><Name>FL3</Name><Origin><Source>GeometricFeature</Source><FeatureName>planar surface 55</FeatureName></Origin><PrimaryAxis><DefinedDirection>+X</DefinedDirection><Source>GeometricFeature</Source><SourceDirection>+Z</SourceDirection><FeatureName>planar surface 55</FeatureName></PrimaryAxis><SecondaryAxis><DefinedDirection>-Y</DefinedDirection><Source>GeometricFeature</Source><SourceDirection>+X</SourceDirection><FeatureName>segment 380</FeatureName></SecondaryAxis></Value></Frame><Frame><Id>Frame10</Id><Value><Name>FL4</Name><Origin><Source>GeometricFeature</Source><FeatureName>planar surface 63</FeatureName></Origin><PrimaryAxis><DefinedDirection>+X</DefinedDirection><Source>GeometricFeature</Source><SourceDirection>+Z</SourceDirection><FeatureName>planar surface 63</FeatureName></PrimaryAxis><SecondaryAxis><DefinedDirection>+Y</DefinedDirection><Source>CenterOfMassFrame</Source><SourceDirection>-Z</SourceDirection><FeatureName></FeatureName></SecondaryAxis></Value></Frame><Frame><Id>Frame11</Id><Value><Name>Frame_SwimArmFL</Name><Origin><Source>GeometricFeature</Source><FeatureName>circular curve 2</FeatureName></Origin><PrimaryAxis><DefinedDirection>+Z</DefinedDirection><Source>GeometricFeature</Source><SourceDirection>+Z</SourceDirection><FeatureName>segment 1</FeatureName></PrimaryAxis><SecondaryAxis><DefinedDirection>-Y</DefinedDirection><Source>ReferenceFrame</Source><SourceDirection>+X</SourceDirection><FeatureName></FeatureName></SecondaryAxis></Value></Frame></Frames>  GraphicType=FromGeometry  MarkerShape=Sphere  MarkerSize=10  GraphicVisPropType=SimpleVisualProperties  GraphicDiffuseColor=[0.5 0.5 0.5]  GraphicSpecularColor=[0.5 0.5 0.5 1.0]  GraphicAmbientColor=[0.15 0.15 0.15 1.0]  GraphicEmissiveColor=[0.0 0.0 0.0 1.0]  GraphicShininess=75  GraphicOpacity=1.0  GeometryShape=FromFile  RectangleSize=[1 1]  RectangleSizeUnits=m  BrickDimensions=[1 1 1]  BrickDimensionUnits=m  CylinderRadius=1  CylinderRadiusUnits=m  CylinderLength=1  CylinderLengthUnits=m  SphereRadius=1  SphereRadiusUnits=m  EllipsoidRadii=[1 1 1]  EllipsoidRadiiUnits=m  ExtrusionCrossSection=[1 1; -1 1; -1 -1; 1 -1]  ExtrusionCrossSectionUnits=m  ExtrusionLength=1  ExtrusionLengthUnits=m  PolygonNumSides=3  PolygonOuterRadius=1  PolygonOuterRadiusUnits=m  ExtGeomFileType=STEP  ExtGeomFileName=D:\FSEC\Matlab\Chasis\STP\Frame.stp  ExtGeomFileUnits=m  RevolutionCrossSection=[1 1; 1 -1; 2 -1; 2 1]  RevolutionCrossSectionUnits=m  RevolutionExtent=Full  RevolutionAngle=180  RevolutionAngleUnits=deg
  Mechanism Configuration : sm_lib/Utilities/Mechanism Configuration  UniformGravity=Constant  GravityVector=[0 0 -9.8]  GravityUnits=m/s^2  LinearizationDelta=0.001
  PS-Simulink Converter : nesl_utility/PS-Simulink Converter  PhysicalDomain=network_engine_domain  SubClassName=ps_output  LeftPortType=input  RightPortType=output  PseudoPeriodic=off  Frequencies=[]  Unit=N  AffineConversion=off
  PS-Simulink Converter1 : nesl_utility/PS-Simulink Converter  PhysicalDomain=network_engine_domain  SubClassName=ps_output  LeftPortType=input  RightPortType=output  PseudoPeriodic=off  Frequencies=[]  Unit=N*m  AffineConversion=off
  PS-Simulink Converter2 : nesl_utility/PS-Simulink Converter  PhysicalDomain=network_engine_domain  SubClassName=ps_output  LeftPortType=input  RightPortType=output  PseudoPeriodic=off  Frequencies=[]  Unit=1  AffineConversion=off
  Reference Frame{,1..5} (6 alike) : sm_lib/Frames and Transforms/Reference Frame
  Rigid Transform : sm_lib/Frames and Transforms/Rigid Transform  TranslationMethod=Cartesian  TranslationStandardOffset=0  TranslationLengthUnit=mm  TranslationStandardAxis=+Z  TranslationCartesianOffset=[-659.4 0 0]  TranslationROffset=0  TranslationROffsetUnits=m  TranslationZOffset=0  TranslationZOffsetUnits=m  TranslationThetaOffset=0  TranslationThetaOffsetUnits=deg  RotationMethod=None  RotationAngleUnits=deg  RotationStandardAxis=+Z  RotationAngle=0.0  RotationArbitraryAxis=[0 0 1]  FollAlignAxisA=+X  BaseAlignAxisA=+Y  FollAlignAxisB=+Y  BaseAlignAxisB=+Z  RotationSequenceAxes=FollowerAxes  RotationSequence=XYX  RotationSequenceAngles=[0 0 0]  RotationSequenceAnglesUnits=deg  RotationMatrix=[1 0 0; 0 1 0; 0 0 1]
  Selector : Selector  InputPortWidth=3  IndexOptions=Index vector (dialog)  Indices=1  OutputSizes=1
  Selector1 : Selector  InputPortWidth=3  IndexOptions=Index vector (dialog)  Indices=2  OutputSizes=1
  Selector2 : Selector  InputPortWidth=3  IndexOptions=Index vector (dialog)  Indices=3  OutputSizes=1
  Simulink-PS Converter : nesl_utility/Simulink-PS Converter  PhysicalDomain=network_engine_domain  SubClassName=ps_input  LeftPortType=input  RightPortType=output  PseudoPeriodic=off  Frequencies=[]  NoiseDistribution=none  NoiseParameters=[]  Unit=N  AffineConversion=off  FilteringAndDerivatives=provide  SimscapeFilterOrder=1  InputFilterTimeConstant=0.001  UdotUserProvided=0
  Simulink-PS Converter1 : nesl_utility/Simulink-PS Converter  PhysicalDomain=network_engine_domain  SubClassName=ps_input  LeftPortType=input  RightPortType=output  PseudoPeriodic=off  Frequencies=[]  NoiseDistribution=none  NoiseParameters=[]  Unit=N  AffineConversion=off  FilteringAndDerivatives=provide  SimscapeFilterOrder=1  InputFilterTimeConstant=0.001  UdotUserProvided=0
  Simulink-PS Converter2 : nesl_utility/Simulink-PS Converter  PhysicalDomain=network_engine_domain  SubClassName=ps_input  LeftPortType=input  RightPortType=output  PseudoPeriodic=off  Frequencies=[]  NoiseDistribution=none  NoiseParameters=[]  Unit=N  AffineConversion=off  FilteringAndDerivatives=provide  SimscapeFilterOrder=1  InputFilterTimeConstant=0.001  UdotUserProvided=0
  Solver Configuration : nesl_utility/Solver Configuration  PhysicalDomain=network_engine_domain  SubClassName=solver  LeftPortType=input  RightPortType=generic  Tones=[]  Harmonics=[]  SimulateNoise=off  Profile=off  UseLocalSampling=off  EnableSwitchedLinearOptims=on  FrequencyDomain=off  UseCCode=off  RelTol=0.001  AbsTol=1e-06  MinStep=1e-09  ToWorkspace=off  RevertToSquareIcSolve=off  NumHomotopyIterations=100  PhasorMode=off  PhasorModeNumHarmonics=1  DoDC=off  ResidualTolerance=1e-09  UseLocalSolver=off  LocalSolverChoice=NE_BACKWARD_EULER_ADVANCER  LocalSolverSampleTime=0.001  DoFixedCost=off  MaxNonlinIter=3  MaxModeIter=2  LinearAlgebra=Sparse  EquationFormulation=NE_TIME_EF  DelaysMemoryBudget=1024  AutomaticFiltering=on  FilteringTimeConstant=0.001
  Terminator : Terminator
  Terminator1 : Terminator
  Transform Sensor : sm_lib/Frames and Transforms/Transform Sensor  MeasurementFrame=Base  SenseAngle=off  SenseAxis=on  SenseAngle1=off  SenseAngle2=off  SenseAngle3=off  SenseQ=off  SenseR=off  SenseOmegaX=off  SenseOmegaY=off  SenseOmegaZ=off  SenseOmega1=off  SenseOmega2=off  SenseOmega3=off  SenseQDot=off  SenseRDot=off  SenseAlphaX=off  SenseAlphaY=off  SenseAlphaZ=off  SenseAlpha1=off  SenseAlpha2=off  SenseAlpha3=off  SenseQDDot=off  SenseRDDot=off  SenseX=off  SenseY=off  SenseZ=off  SenseRad=off  SenseAzim=off  SenseDist=off  SenseInc=off  SenseXDot=off  SenseYDot=off  SenseZDot=off  SenseRadDot=off  SenseAzimDot=off  SenseDistDot=off  SenseIncDot=off  SenseXDDot=off  SenseYDDot=off  SenseZDDot=off  SenseRadDDot=off  SenseAzimDDot=off  SenseDistDDot=off  SenseIncDDot=off
  Transport Delay : TransportDelay  DelayTime=0.02
  Transport Delay1 : TransportDelay  DelayTime=0.02
  Unary Minus : UnaryMinus
  Weld Joint : sm_lib/Joints/Weld Joint  SenseConstraintForce=off  SenseConstraintForceX=off  SenseConstraintForceY=off  SenseConstraintForceZ=off  SenseConstraintTorque=off  SenseConstraintTorqueX=off  SenseConstraintTorqueY=off  SenseConstraintTorqueZ=off  SenseTotalForce=on  SenseTotalForceX=off  SenseTotalForceY=off  SenseTotalForceZ=off  SenseTotalTorque=on  SenseTotalTorqueX=off  SenseTotalTorqueY=off  SenseTotalTorqueZ=off  CompositeWrenchDir=FollowerOnBase  CompositeWrenchFrame=BaseFrame
  World Frame : sm_lib/Frames and Transforms/World Frame
  FWhlsForces : Outport  ConcatenationDimension=1
  FWhlMoments : Outport  Port=2  ConcatenationDimension=1
  Camber : Outport  Port=3  ConcatenationDimension=1
  wires:
  PS-Simulink Converter/1 -> Transport Delay/1
  PS-Simulink Converter1/1 -> Transport Delay1/1
  Selector2/1 -> Unary Minus/1
  Selector/1 -> Simulink-PS Converter1/1
  Selector1/1 -> Simulink-PS Converter/1
  FWhls/1 -> Selector2/1, Selector/1, Selector1/1
  Transport Delay/1 -> FWhlsForces/1
  Transport Delay1/1 -> FWhlMoments/1
  Unary Minus/1 -> Simulink-PS Converter2/1
  PS-Simulink Converter2/1 -> Demux/1
  Demux/1 -> Camber/1
  Demux/3 -> Terminator1/1
  Demux/2 -> Terminator/1
  connections:
  Transform Sensor/LConn1 -- World Frame/RConn1 -- Weld Joint/LConn1 -- Mechanism Configuration/RConn1 -- Solver Configuration/RConn1
  Weld Joint/RConn3 -- PS-Simulink Converter1/LConn1
  Reference Frame3/RConn1 -- Frame/LConn5
  Reference Frame2/RConn1 -- Frame/RConn6
  Reference Frame/RConn1 -- Frame/RConn4
  Weld Joint/RConn2 -- PS-Simulink Converter/LConn1
  FR/LConn6 -- Frame/LConn4
  FR/LConn5 -- Frame/LConn3
  FR/LConn4 -- Frame/LConn2
  FR/LConn2 -- Rigid Transform/LConn1 -- Frame/RConn3
  FR/LConn3 -- Frame/LConn1
  FR/LConn1 -- Frame/RConn2
  Reference Frame4/RConn1 -- Frame/LConn6
  Transform Sensor/RConn1 -- FR/LConn7 -- External Force and Torque/RConn1
  Reference Frame1/RConn1 -- Frame/RConn5
  Simulink-PS Converter/RConn1 -- External Force and Torque/LConn2
  Simulink-PS Converter2/RConn1 -- External Force and Torque/LConn3
  Simulink-PS Converter1/RConn1 -- External Force and Torque/LConn1
  Rigid Transform/RConn1 -- Weld Joint/RConn1
  Frame/RConn1 -- Reference Frame5/RConn1
  PS-Simulink Converter2/LConn1 -- Transform Sensor/RConn2
